simulink model "QuadcopterSimulation"  (R2024a)
settings: Solver=FixedStepAuto  StartTime=0.0  StopTime=inf  FixedStep=SampleTime  RelTol=1e-3
PreLoadFcn:
  | %Based on the quadcopter model used in jMAVSim
  | 
  | Ixx = 0.005; %Kgm^2
  | Iyy = 0.005;
  | Izz = 0.009;
  | 
  | 
  | inertia = diag([Ixx, Iyy, Izz]);
  | 
  | mass = 0.8; %Kg
  | g = 9.81; %m/s^2
  | 
  | armLength = 0.33/2; % length of Arm measured from center in m
  | 
  | rotorThrustMax = 4; %N
  | 
  | rotorTorqueMax = 0.05 %Nm
  | 
  | rotorTimeConst = 0.005 % time constant of rotor (motor + propeller)
  | 
  | %rotorOffset = [0 0 0]; % Rotors position offsets from Gravity center
  | 
  | dragCoeffMov = 0.01; %drag coefficient for linear motion of quadcopter
  | 
  | % Initial states
  | init.posNED = [0, 0, 0]; % m
  | init.vb = [0 0 0]'; %m/s
  | init.euler = [0, 0, 0]'; %Roll Pitch Yaw Rads
  | init.angRates = [0, 0, 0]; %rad/s
  | 
  | 
  | %Computed from above values
  | rotorPositions = zeros(3,4);
  | axisD = armLength/sqrt(2);
  | rotorPositions(:,1) = [axisD, axisD, 0]';
  | rotorPositions(:,2) = [-axisD, -axisD, 0]';
  | rotorPositions(:,3) = [+axisD, -axisD, 0]';
  | rotorPositions(:,4) = [-axisD, axisD, 0]';
  | rotorDir = [-1, -1, 1, 1]; %rotation direction. +ve = clockwise
undefined symbols (not defined in the file): ax, ay, az, Earth, Payload, SampleTime, vx, vy, vz, WGS84, x, y, z
libraries: px4uORBlib x2, aerolibtransform2 x1, uavmavlinklib x1, instrumentlib x1
settings Model: Creator=The MathWorks, Inc.  LastModifiedBy=nate
settings SolverCC: AlgebraicLoopSolver=LineSearch
settings DebuggingCC: UnconnectedInputMsg=warning  UnconnectedOutputMsg=warning  UnconnectedLineMsg=warning
settings ModelReferenceCC: EnableRefExpFcnMdlSchedulingChecks=on
settings RTWCC: GPUComputeCapability=3.5  DLArmComputeVersion=19.05

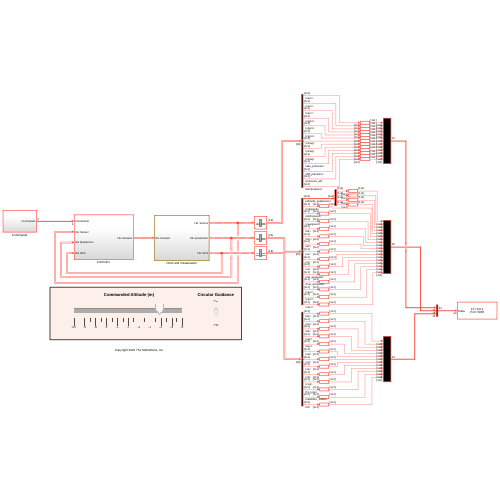
[thumbnail: Simulink's stored preview of the top-level diagram]
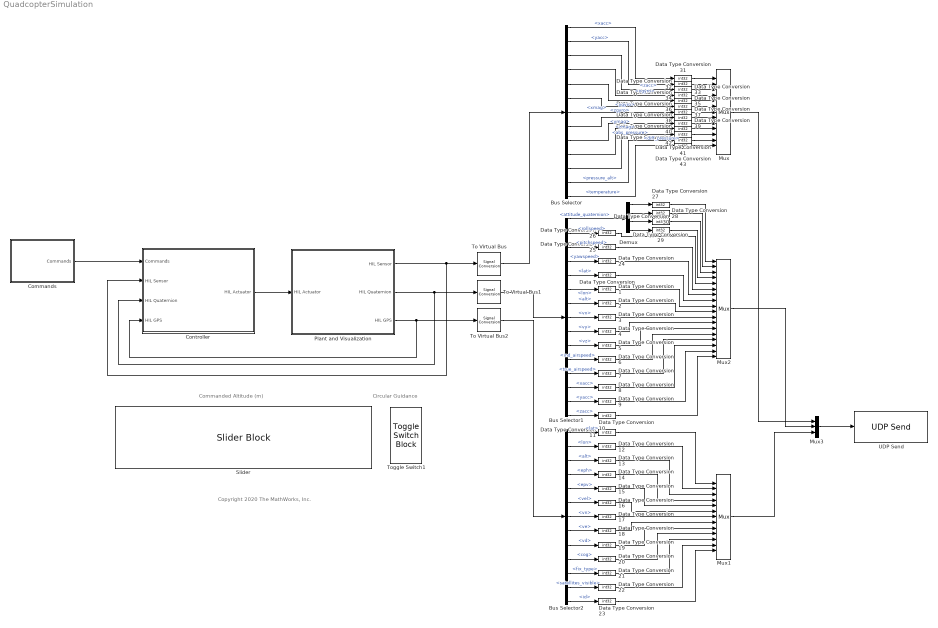
== system QuadcopterSimulation ==
  note: Commanded Altitude (m)
  note: Circular Guidance
  note: Copyright 2020 The MathWorks, Inc.
  Bus Selector : BusSelector  OutputSignals=Payload.xacc,Payload.yacc,Payload.zacc,Payload.xgyro,Payload.ygyro,Payload.zgyro,Payload.xmag,Payload.ymag,Payload.zmag,Payload.abs_pressure,Payload.diff_pressure,Payload.pressure_alt,Payload.temperature
  Bus Selector1 : BusSelector  OutputSignals=Payload.attitude_quaternion,Payload.rollspeed,Payload.pitchspeed,Payload.yawspeed,Payload.lat,Payload.lon,Payload.alt,Payload.vx,Payload.vy,Payload.vz,Payload.ind_airspeed,Payload.true_airspeed,Payload.xacc,Payload.yacc,Payload.zacc
  Bus Selector2 : BusSelector  OutputSignals=Payload.lat,Payload.lon,Payload.alt,Payload.eph,Payload.epv,Payload.vel,Payload.vn,Payload.ve,Payload.vd,Payload.cog,Payload.fix_type,Payload.satellites_visible,Payload.id
  Commands : Subsystem
  "Controller " : Subsystem
  Data Type Conversion{,1..43} (44 alike) : DataTypeConversion  OutDataTypeStr=int32  SaturateOnIntegerOverflow=off
  Demux : Demux
  Mux : Mux  Inputs=13
  Mux1 : Mux  Inputs=13
  Mux2 : Mux  Inputs=18
  Mux3 : Mux  Inputs=3
  Plant and Visualization : Subsystem
  Slider : SliderBlock  LabelPosition=Hide  ScaleMin=-10  ScaleMax=0  TickInterval=1
  To Virtual Bus : SignalConversion  ConversionOutput=Virtual bus  OverrideOpt=off
  To Virtual Bus1 : SignalConversion  ConversionOutput=Virtual bus  OverrideOpt=off
  To Virtual Bus2 : SignalConversion  ConversionOutput=Virtual bus  OverrideOpt=off
  Toggle Switch1 : ToggleSwitchBlock  LabelPosition=Hide
      settings: Values={{'Off', 'On'}, [0 1]}
  UDP Send : instrumentlib/UDP Send  Host=127.0.0.1  Port=5005  LocalAddress=0.0.0.0  LocalPort=-1  EnablePortSharing=off  OutputDatagramPacketSize=1024  ByteOrder=little-endian  EnableBlockingMode=on  SimulateUsing=Interpreted execution
  wires:
  Commands/1(Commands) -> "Controller "/1(Commands)
  "Controller "/1(HIL Actuator) -> Plant and Visualization/1(HIL Actuator)
  Plant and Visualization/1(HIL Sensor) -> To Virtual Bus/1, "Controller "/2(HIL Sensor)
  Plant and Visualization/2(HIL Quaternion) -> To Virtual Bus1/1, "Controller "/3(HIL Quaternion)
  Plant and Visualization/3(HIL GPS) -> To Virtual Bus2/1, "Controller "/4(HIL GPS)
  To Virtual Bus/1 -> Bus Selector/1
  To Virtual Bus1/1 -> Bus Selector1/1
  To Virtual Bus2/1 -> Bus Selector2/1
  Bus Selector1/1 -> Demux/1  "<attitude_quaternion>"
  Bus Selector/1 -> Data Type Conversion31/1  "<xacc>"
  Bus Selector/2 -> Data Type Conversion32/1  "<yacc>"
  Bus Selector/3 -> Data Type Conversion33/1  "<zacc>"
  Bus Selector/4 -> Data Type Conversion34/1  "<xgyro>"
  Bus Selector/5 -> Data Type Conversion35/1  "<ygyro>"
  Bus Selector/6 -> Data Type Conversion36/1  "<zgyro>"
  Bus Selector/7 -> Data Type Conversion37/1  "<xmag>"
  Bus Selector/8 -> Data Type Conversion38/1  "<ymag>"
  Bus Selector/9 -> Data Type Conversion39/1  "<zmag>"
  Bus Selector/10 -> Data Type Conversion40/1  "<abs_pressure>"
  Bus Selector/11 -> Data Type Conversion41/1  "<diff_pressure>"
  Bus Selector/12 -> Data Type Conversion42/1  "<pressure_alt>"
  Bus Selector/13 -> Data Type Conversion43/1  "<temperature>"
  Bus Selector2/13 -> Data Type Conversion23/1  "<id>"
  Bus Selector2/12 -> Data Type Conversion22/1  "<satellites_visible>"
  Bus Selector2/11 -> Data Type Conversion21/1  "<fix_type>"
  Bus Selector2/10 -> Data Type Conversion20/1  "<cog>"
  Bus Selector2/9 -> Data Type Conversion19/1  "<vd>"
  Bus Selector2/8 -> Data Type Conversion18/1  "<ve>"
  Bus Selector2/7 -> Data Type Conversion17/1  "<vn>"
  Bus Selector2/6 -> Data Type Conversion16/1  "<vel>"
  Bus Selector2/5 -> Data Type Conversion15/1  "<epv>"
  Bus Selector2/4 -> Data Type Conversion14/1  "<eph>"
  Bus Selector2/3 -> Data Type Conversion13/1  "<alt>"
  Bus Selector2/2 -> Data Type Conversion12/1  "<lon>"
  Bus Selector2/1 -> Data Type Conversion11/1  "<lat>"
  Demux/1 -> Data Type Conversion27/1
  Demux/2 -> Data Type Conversion28/1
  Demux/3 -> Data Type Conversion29/1
  Demux/4 -> Data Type Conversion30/1
  Bus Selector1/2 -> Data Type Conversion26/1  "<rollspeed>"
  Bus Selector1/3 -> Data Type Conversion25/1  "<pitchspeed>"
  Bus Selector1/4 -> Data Type Conversion24/1  "<yawspeed>"
  Bus Selector1/5 -> Data Type Conversion/1  "<lat>"
  Bus Selector1/6 -> Data Type Conversion1/1  "<lon>"
  Bus Selector1/7 -> Data Type Conversion2/1  "<alt>"
  Bus Selector1/8 -> Data Type Conversion3/1  "<vx>"
  Bus Selector1/9 -> Data Type Conversion4/1  "<vy>"
  Bus Selector1/10 -> Data Type Conversion5/1  "<vz>"
  Bus Selector1/11 -> Data Type Conversion6/1  "<ind_airspeed>"
  Bus Selector1/12 -> Data Type Conversion7/1  "<true_airspeed>"
  Bus Selector1/13 -> Data Type Conversion8/1  "<xacc>"
  Bus Selector1/14 -> Data Type Conversion9/1  "<yacc>"
  Bus Selector1/15 -> Data Type Conversion10/1  "<zacc>"
  Mux/1 -> Mux3/1
  Mux2/1 -> Mux3/2
  Mux1/1 -> Mux3/3
  Mux3/1 -> UDP Send/1
  Data Type Conversion/1 -> Mux2/8
  Data Type Conversion1/1 -> Mux2/9
  Data Type Conversion2/1 -> Mux2/10
  Data Type Conversion3/1 -> Mux2/11
  Data Type Conversion4/1 -> Mux2/12
  Data Type Conversion5/1 -> Mux2/13
  Data Type Conversion6/1 -> Mux2/14
  Data Type Conversion7/1 -> Mux2/15
  Data Type Conversion8/1 -> Mux2/16
  Data Type Conversion9/1 -> Mux2/17
  Data Type Conversion10/1 -> Mux2/18
  Data Type Conversion11/1 -> Mux1/1
  Data Type Conversion12/1 -> Mux1/2
  Data Type Conversion13/1 -> Mux1/3
  Data Type Conversion14/1 -> Mux1/4
  Data Type Conversion15/1 -> Mux1/5
  Data Type Conversion16/1 -> Mux1/6
  Data Type Conversion17/1 -> Mux1/7
  Data Type Conversion18/1 -> Mux1/8
  Data Type Conversion19/1 -> Mux1/9
  Data Type Conversion20/1 -> Mux1/10
  Data Type Conversion21/1 -> Mux1/11
  Data Type Conversion22/1 -> Mux1/12
  Data Type Conversion23/1 -> Mux1/13
  Data Type Conversion24/1 -> Mux2/7
  Data Type Conversion25/1 -> Mux2/6
  Data Type Conversion26/1 -> Mux2/5
  Data Type Conversion27/1 -> Mux2/1
  Data Type Conversion28/1 -> Mux2/2
  Data Type Conversion29/1 -> Mux2/3
  Data Type Conversion30/1 -> Mux2/4
  Data Type Conversion31/1 -> Mux/1
  Data Type Conversion32/1 -> Mux/2
  Data Type Conversion33/1 -> Mux/3
  Data Type Conversion34/1 -> Mux/4
  Data Type Conversion35/1 -> Mux/5
  Data Type Conversion36/1 -> Mux/6
  Data Type Conversion37/1 -> Mux/7
  Data Type Conversion38/1 -> Mux/8
  Data Type Conversion39/1 -> Mux/9
  Data Type Conversion40/1 -> Mux/10
  Data Type Conversion41/1 -> Mux/11
  Data Type Conversion42/1 -> Mux/12
  Data Type Conversion43/1 -> Mux/13

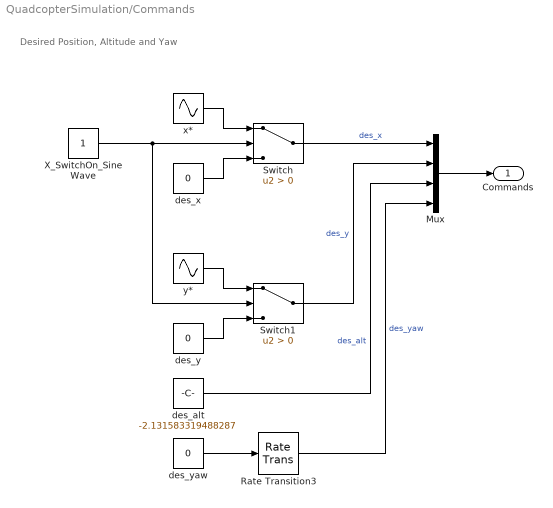
== system QuadcopterSimulation/Commands ==
  note: Desired Position, Altitude and Yaw
  Mux : Mux
  Rate Transition3 : RateTransition  OutPortSampleTime=SampleTime
  Switch : Switch  Criteria=u2 > Threshold  SaturateOnIntegerOverflow=off  InputSameDT=off
  Switch1 : Switch  Criteria=u2 > Threshold  SaturateOnIntegerOverflow=off  InputSameDT=off
  X_SwitchOn_Sine Wave : Constant  SampleTime=SampleTime
  des_alt : Constant  Value=-2.131583319488287  SampleTime=SampleTime
  des_x : Constant  Value=0  SampleTime=SampleTime
  des_y : Constant  Value=0  SampleTime=SampleTime
  des_yaw : Constant  Value=0  SampleTime=SampleTime
  x* : Sin  Frequency=2*pi*.125  Phase=-pi/2  Samples=10000  SampleTime=SampleTime
  y* : Sin  Frequency=2*pi*.125  Samples=10000  SampleTime=SampleTime
  Commands : Outport
  wires:
  Rate Transition3/1 -> Mux/4  "des_yaw"
  des_x/1 -> Switch/3
  Switch/1 -> Mux/1  "des_x"
  Switch1/1 -> Mux/2  "des_y"
  X_SwitchOn_Sine Wave/1 -> Switch1/2, Switch/2
  des_yaw/1 -> Rate Transition3/1
  y*/1 -> Switch1/1
  des_y/1 -> Switch1/3
  x*/1 -> Switch/1
  Mux/1 -> Commands/1
  des_alt/1 -> Mux/3  "des_alt"

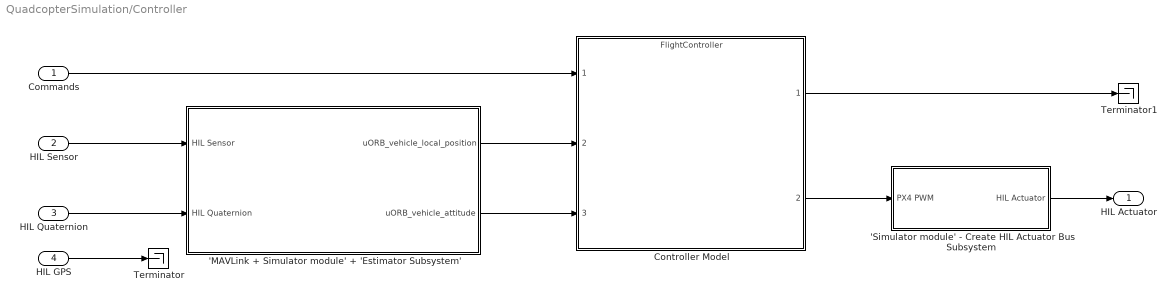
== system QuadcopterSimulation/Controller  ==
  Commands : Inport
  HIL Sensor : Inport  Port=2
  HIL Quaternion : Inport  Port=3
  HIL GPS : Inport  Port=4
  'MAVLink + Simulator module' + 'Estimator Subsystem' : Subsystem
      settings: PortSchema="{\"entries\":[{\"content\":{\"sides\":[{\"content\":{\"connectorIds\":[]},\"type\":\"ConnectorPlacement.EquallySpacedRectSide\",\"uuid\":\"18f19b7f-7de0-4ac4-a24f-d8ceb747f924\"},{\"content\":{\"connectorIds\":[],\"side\":\"RIGHT\"},\"type\":\"ConnectorPlacement.EquallySpacedRectSide\",\"uuid\":\"b474fbae-f8e2-4c2b-be96-a63ee47992dd\"},{\"content\":{\"connectorIds\":[\"In1\",\"In2\"],\"side\":\"TOP\"},\"type\":\"ConnectorPlacement.EquallySpacedRectSide\",\"uuid\":\"67540526-de5d-4152-a323-fd05419e6390\"},{\"content\":{\"connectorIds\":[\"Out1\",\"Out2\"],\"side\":\"BOTTOM\"},\"type\":\"ConnectorPlacement.EquallySpacedRectSide\",\"uuid\":\"c51ef1bd-db79-4835-87f1-e9dccd8fce9f\"},{\"content\":{\"connectorIds\":[],\"side\":\"HIDDEN\"},\"type\":\"ConnectorPlacement.EquallySpacedRectSide\",\"uuid\":\"82a3913e-38ee-407a-aef4-9df458d840d7\"}]},\"type\":\"ConnectorPlacement.EquallySpacedConnector\",\"uuid\":\"5015a705-00cf-433b-8716-d3e1ebe8eda0\"}],\"packageUris\":[\"http://schema.mathworks.com/mf0/Connector/R2020b\"],\"version\":\"1.0\"}"
  'Simulator module' - Create HIL Actuator Bus Subsystem : Subsystem
  Controller Model : ModelReference  ModelNameDialog=FlightController.slx  SimulationMode=Normal  ModelReferenceVersion=8.0
  Terminator : Terminator
  Terminator1 : Terminator
  HIL Actuator : Outport
  wires:
  Controller Model/2 -> 'Simulator module' - Create HIL Actuator Bus Subsystem/1(PX4 PWM)
  'Simulator module' - Create HIL Actuator Bus Subsystem/1(HIL Actuator) -> HIL Actuator/1
  HIL Sensor/1 -> 'MAVLink + Simulator module' + 'Estimator Subsystem'/2(HIL Sensor)
  HIL Quaternion/1 -> 'MAVLink + Simulator module' + 'Estimator Subsystem'/1(HIL Quaternion)
  Commands/1 -> Controller Model/1
  'MAVLink + Simulator module' + 'Estimator Subsystem'/2(uORB_vehicle_local_position) -> Controller Model/2
  'MAVLink + Simulator module' + 'Estimator Subsystem'/1(uORB_vehicle_attitude) -> Controller Model/3
  HIL GPS/1 -> Terminator/1
  Controller Model/1 -> Terminator1/1

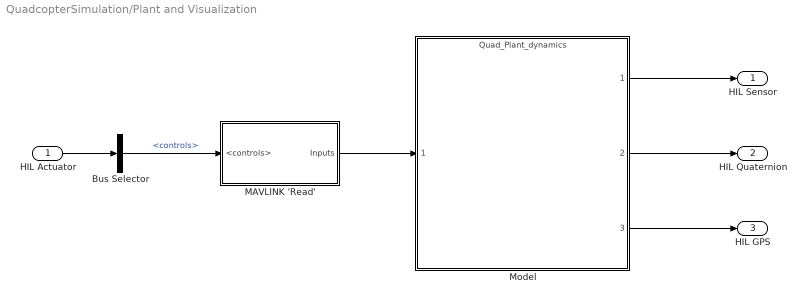
== system QuadcopterSimulation/Plant and Visualization ==
  HIL Actuator : Inport
  Bus Selector : BusSelector  OutputSignals=Payload.controls
  MAVLINK 'Read' : Subsystem
  Model : ModelReference  ModelNameDialog=Quad_Plant_dynamics.slx  SimulationMode=Normal  ModelReferenceVersion=8.1
  HIL Sensor : Outport
  HIL Quaternion : Outport  Port=2
  HIL GPS : Outport  Port=3
  wires:
  HIL Actuator/1 -> Bus Selector/1
  Bus Selector/1 -> MAVLINK 'Read'/1(<controls>)  "<controls>"
  MAVLINK 'Read'/1(Inputs) -> Model/1
  Model/1 -> HIL Sensor/1
  Model/2 -> HIL Quaternion/1
  Model/3 -> HIL GPS/1

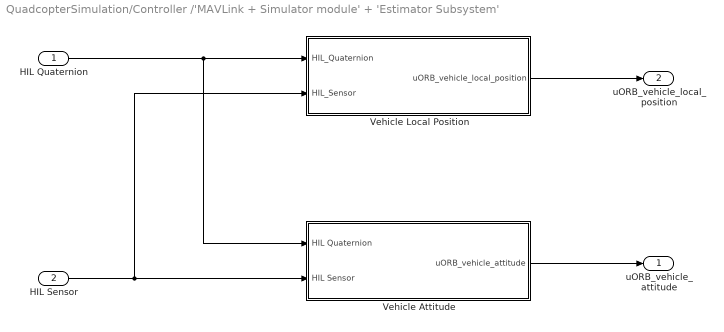
== system QuadcopterSimulation/Controller /'MAVLink + Simulator module' + 'Estimator Subsystem' ==
  HIL Quaternion : Inport
  HIL Sensor : Inport  Port=2
  Vehicle Attitude : Subsystem
  Vehicle Local Position : Subsystem
  uORB_vehicle_attitude : Outport
  uORB_vehicle_local_position : Outport  Port=2
  wires:
  HIL Quaternion/1 -> Vehicle Attitude/1(HIL Quaternion), Vehicle Local Position/1(HIL_Quaternion)
  HIL Sensor/1 -> Vehicle Local Position/2(HIL_Sensor), Vehicle Attitude/2(HIL Sensor)
  Vehicle Local Position/1(uORB_vehicle_local_position) -> uORB_vehicle_local_position/1
  Vehicle Attitude/1(uORB_vehicle_attitude) -> uORB_vehicle_attitude/1

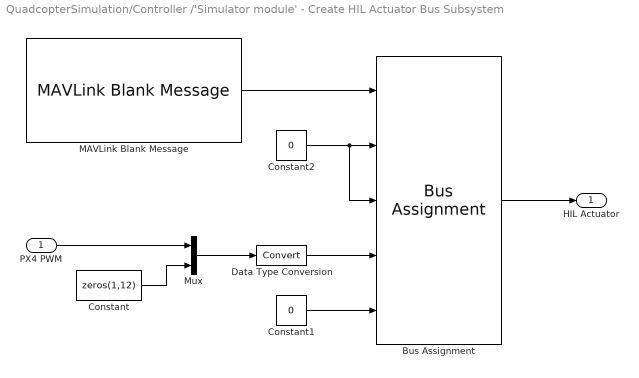
== system QuadcopterSimulation/Controller /'Simulator module' - Create HIL Actuator Bus Subsystem ==
  PX4 PWM : Inport
  Bus Assignment : BusAssignment  AssignedSignals=Payload.time_usec,Payload.flags,Payload.controls,Payload.mode
  Constant : Constant  Value=zeros(1,12)  OutDataTypeStr=Inherit: Inherit via back propagation  SampleTime=SampleTime
  Constant1 : Constant  Value=0  OutDataTypeStr=Inherit: Inherit via back propagation  SampleTime=SampleTime
  Constant2 : Constant  Value=0  OutDataTypeStr=Inherit: Inherit via back propagation  SampleTime=SampleTime
  Data Type Conversion : DataTypeConversion  SaturateOnIntegerOverflow=off  RndMeth=Floor
  MAVLink Blank Message : uavmavlinklib/MAVLink Blank Message  dialectSource=Select from standard MAVLink dialects  dialect=common.xml  dialectCustom=common.xml  version=2  messageType=HIL_ACTUATOR_CONTROLS  SystemID=1  ComponentID=1  SampleTime=SampleTime
  Mux : Mux  Inputs=2
  HIL Actuator : Outport
  wires:
  MAVLink Blank Message/1 -> Bus Assignment/1
  Bus Assignment/1 -> HIL Actuator/1
  PX4 PWM/1 -> Mux/1
  Constant/1 -> Mux/2
  Mux/1 -> Data Type Conversion/1
  Constant2/1 -> Bus Assignment/3, Bus Assignment/2
  Constant1/1 -> Bus Assignment/5
  Data Type Conversion/1 -> Bus Assignment/4

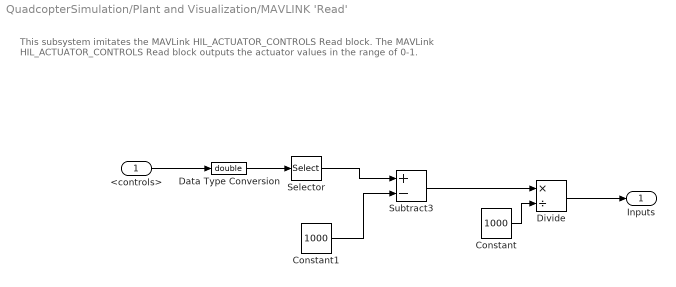
== system QuadcopterSimulation/Plant and Visualization/MAVLINK 'Read' ==
  note: This subsystem imitates the MAVLink HIL_ACTUATOR_CONTROLS Read block. The MAVLink HIL_ACTUATOR_CONTROLS Read block outputs the
      | actuator values in the range of 0-1.
  <controls> : Inport
  Constant : Constant  Value=1000  SampleTime=SampleTime
  Constant1 : Constant  Value=1000  OutDataTypeStr=Inherit: Inherit via back propagation  SampleTime=SampleTime
  Data Type Conversion : DataTypeConversion  OutDataTypeStr=double  SaturateOnIntegerOverflow=off  RndMeth=Floor
  Divide : Product  Inputs=*/
  Selector : Selector  InputPortWidth=16  IndexOptions=Index vector (dialog)  Indices=[1:4]  OutputSizes=1
  Subtract3 : Sum  Inputs=+-
  Inputs : Outport
  wires:
  <controls>/1 -> Data Type Conversion/1
  Constant/1 -> Divide/2
  Data Type Conversion/1 -> Selector/1
  Constant1/1 -> Subtract3/2
  Subtract3/1 -> Divide/1
  Selector/1 -> Subtract3/1
  Divide/1 -> Inputs/1

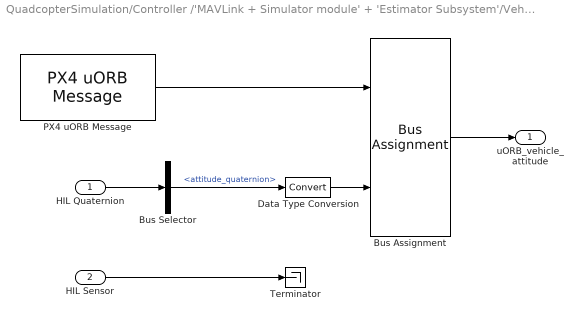
== system QuadcopterSimulation/Controller /'MAVLink + Simulator module' + 'Estimator Subsystem'/Vehicle Attitude ==
  HIL Quaternion : Inport
  HIL Sensor : Inport  Port=2
  Bus Assignment : BusAssignment  AssignedSignals=q
  Bus Selector : BusSelector  OutputSignals=Payload.attitude_quaternion
  Data Type Conversion : DataTypeConversion  SaturateOnIntegerOverflow=off  RndMeth=Floor
  PX4 uORB Message : px4uORBlib/PX4 uORB Message  uORBTopic=VehicleAttitude  SampleTime=SampleTime  selectInstance=vehicle_attitude
  Terminator : Terminator
  uORB_vehicle_attitude : Outport
  wires:
  HIL Quaternion/1 -> Bus Selector/1
  Data Type Conversion/1 -> Bus Assignment/2
  PX4 uORB Message/1 -> Bus Assignment/1
  Bus Assignment/1 -> uORB_vehicle_attitude/1
  HIL Sensor/1 -> Terminator/1
  Bus Selector/1 -> Data Type Conversion/1  "<attitude_quaternion>"

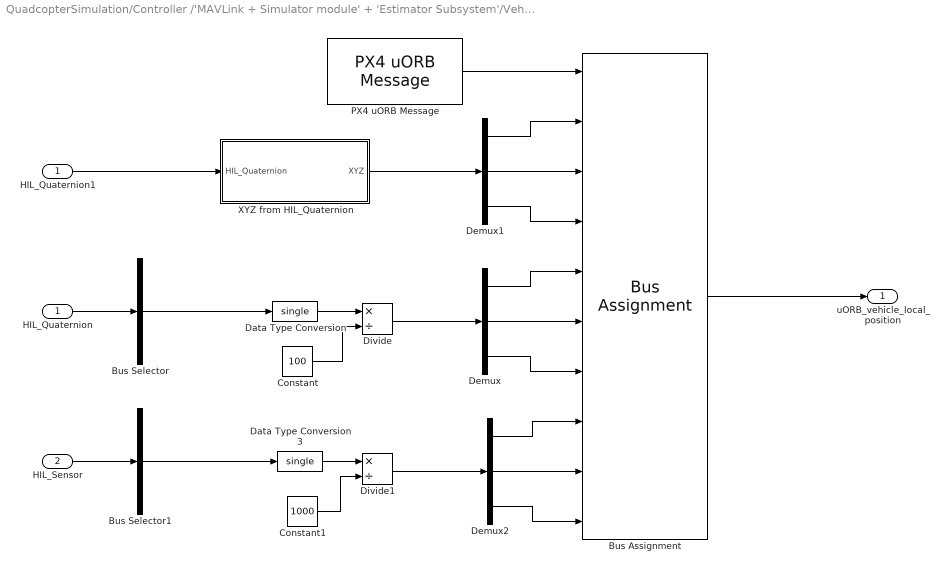
== system QuadcopterSimulation/Controller /'MAVLink + Simulator module' + 'Estimator Subsystem'/Vehicle Local Position ==
  HIL_Quaternion : Inport
  HIL_Sensor : Inport  Port=2
  Bus Assignment : BusAssignment  AssignedSignals=x,y,z,vx,vy,vz,ax,ay,az
  Bus Selector : BusSelector  OutputSignals=Payload.vx,Payload.vy,Payload.vz  OutputAsBus=on
  Bus Selector1 : BusSelector  OutputSignals=Payload.xacc,Payload.yacc,Payload.zacc  OutputAsBus=on
  Constant : Constant  Value=100  OutDataTypeStr=single  SampleTime=SampleTime
  Constant1 : Constant  Value=1000  OutDataTypeStr=single  SampleTime=SampleTime
  Data Type Conversion : DataTypeConversion  OutDataTypeStr=single  SaturateOnIntegerOverflow=off  RndMeth=Floor
  Data Type Conversion3 : DataTypeConversion  OutDataTypeStr=single  SaturateOnIntegerOverflow=off  RndMeth=Floor
  Demux : Demux  Outputs=3
  Demux1 : Demux  Outputs=3
  Demux2 : Demux  Outputs=3
  Divide : Product  Inputs=*/
  Divide1 : Product  Inputs=*/
  HIL_Quaternion1 : InportShadow
  PX4 uORB Message : px4uORBlib/PX4 uORB Message  uORBTopic=VehicleLocalPosition  SampleTime=SampleTime  selectInstance=vehicle_local_position
  XYZ from HIL_Quaternion : Subsystem
  uORB_vehicle_local_position : Outport
  wires:
  Bus Assignment/1 -> uORB_vehicle_local_position/1
  PX4 uORB Message/1 -> Bus Assignment/1
  Demux/3 -> Bus Assignment/7
  Bus Selector/1 -> Data Type Conversion/1
  Demux/1 -> Bus Assignment/5
  Demux/2 -> Bus Assignment/6
  Demux1/3 -> Bus Assignment/4
  Demux1/1 -> Bus Assignment/2
  Demux1/2 -> Bus Assignment/3
  Data Type Conversion/1 -> Divide/1
  HIL_Quaternion/1 -> Bus Selector/1
  Divide/1 -> Demux/1
  Constant/1 -> Divide/2
  Demux2/2 -> Bus Assignment/9
  Demux2/1 -> Bus Assignment/8
  Demux2/3 -> Bus Assignment/10
  Divide1/1 -> Demux2/1
  Bus Selector1/1 -> Data Type Conversion3/1
  HIL_Sensor/1 -> Bus Selector1/1
  Data Type Conversion3/1 -> Divide1/1
  Constant1/1 -> Divide1/2
  HIL_Quaternion1/1 -> XYZ from HIL_Quaternion/1(HIL_Quaternion)
  XYZ from HIL_Quaternion/1(XYZ) -> Demux1/1

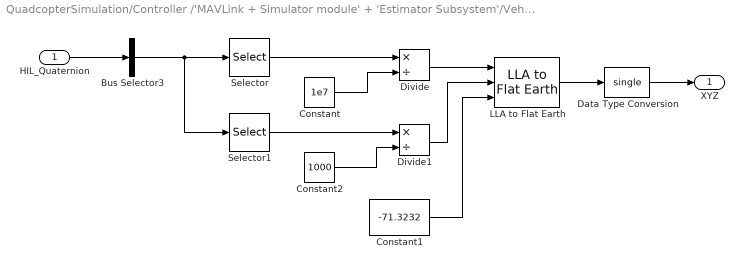
== system QuadcopterSimulation/Controller /'MAVLink + Simulator module' + 'Estimator Subsystem'/Vehicle Local Position/XYZ from HIL_Quaternion ==
  HIL_Quaternion : Inport
  Bus Selector3 : BusSelector  OutputSignals=Payload.lat,Payload.lon,Payload.alt  OutputAsBus=on
  Constant : Constant  Value=1e7  OutDataTypeStr=double
  Constant1 : Constant  Value=-71.3232  OutDataTypeStr=double
  Constant2 : Constant  Value=1000  OutDataTypeStr=double
  Data Type Conversion : DataTypeConversion  OutDataTypeStr=single  SaturateOnIntegerOverflow=off  RndMeth=Floor
  Divide : Product  Inputs=*/
  Divide1 : Product  Inputs=*/
  LLA to Flat Earth : aerolibtransform2/LLA to Flat Earth  units=Metric (MKS)  ptype=Earth (WGS84)  F=1/298.257223563  R=6378137  refPosPort=off  LL0=[0 10]  psi=0
  Selector : Selector  InputPortWidth=3  IndexOptions=Index vector (dialog)  Indices=[1:2]  OutputSizes=1
  Selector1 : Selector  InputPortWidth=3  IndexOptions=Index vector (dialog)  Indices=[3]  OutputSizes=1
  XYZ : Outport
  wires:
  HIL_Quaternion/1 -> Bus Selector3/1
  Constant1/1 -> LLA to Flat Earth/3
  Constant/1 -> Divide/2
  Bus Selector3/1 -> Selector1/1, Selector/1
  Selector/1 -> Divide/1
  Constant2/1 -> Divide1/2
  Selector1/1 -> Divide1/1
  Divide/1 -> LLA to Flat Earth/1
  Divide1/1 -> LLA to Flat Earth/2
  LLA to Flat Earth/1 -> Data Type Conversion/1
  Data Type Conversion/1 -> XYZ/1
